simulink model "Kin3R_Giaitich"  (R2018b)
settings: Solver=VariableStepAuto  StartTime=0.0  StopTime=15  RelTol=1e-3
settings Model: Creator=ADMIN  LastModifiedBy=ADMIN

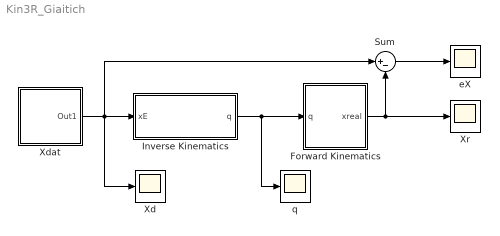
== system Kin3R_Giaitich ==
  Forward Kinematics : Subsystem
  Inverse Kinematics : Subsystem
  Sum : Sum  Inputs=|+-
  Xd : Scope
  Xdat : Subsystem
  Xr : Scope
  eX : Scope
  q : Scope
  wires:
  Xdat/1(Out1) -> Xd/1, Sum/1, Inverse Kinematics/1(xE)
  Inverse Kinematics/1(q) -> q/1, Forward Kinematics/1(q)
  Sum/1 -> eX/1
  Forward Kinematics/1(xreal) -> Xr/1, Sum/2

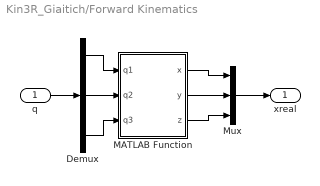
== system Kin3R_Giaitich/Forward Kinematics ==
  q : Inport
  Demux : Demux  Outputs=3
  MATLAB Function : MATLAB Function  TreatAsAtomicUnit=on
  Mux : Mux  Inputs=3
  xreal : Outport
  wires:
  Mux/1 -> xreal/1
  MATLAB Function/2(y) -> Mux/2
  MATLAB Function/1(x) -> Mux/1
  MATLAB Function/3(z) -> Mux/3
  q/1 -> Demux/1
  Demux/3 -> MATLAB Function/3(q3)
  Demux/2 -> MATLAB Function/2(q2)
  Demux/1 -> MATLAB Function/1(q1)

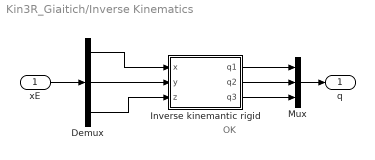
== system Kin3R_Giaitich/Inverse Kinematics ==
  note: OK
  xE : Inport
  Demux : Demux  Outputs=3
  Inverse kinemantic rigid : MATLAB Function  TreatAsAtomicUnit=on
  Mux : Mux  Inputs=3
  q : Outport
  wires:
  Mux/1 -> q/1
  Demux/1 -> Inverse kinemantic rigid/1(x)
  Demux/2 -> Inverse kinemantic rigid/2(y)
  Inverse kinemantic rigid/1(q1) -> Mux/1
  Inverse kinemantic rigid/2(q2) -> Mux/2
  xE/1 -> Demux/1
  Demux/3 -> Inverse kinemantic rigid/3(z)
  Inverse kinemantic rigid/3(q3) -> Mux/3

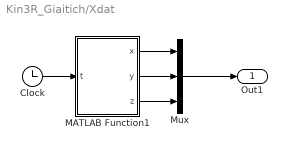
== system Kin3R_Giaitich/Xdat ==
  Clock : Clock
  MATLAB Function1 : MATLAB Function  TreatAsAtomicUnit=on
  Mux : Mux  Inputs=3
  Out1 : Outport
  wires:
  Clock/1 -> MATLAB Function1/1(t)
  Mux/1 -> Out1/1
  MATLAB Function1/1(x) -> Mux/1
  MATLAB Function1/2(y) -> Mux/2
  MATLAB Function1/3(z) -> Mux/3

== matlab function Kin3R_Giaitich/Inverse Kinematics/Inverse kinemantic rigid ==
  data: x input; q1 output; y input; q2 output; z input; q3 output
function [q1,q2,q3] = fcn(x,y,z)
%
[d1,a2,a3]=parameter();
%
q1=atan2(y,x);
%
A3=(x^2+y^2+(d1-z)^2-a2^2-a3^2)/(2*a2*a3);
q3=-acos(A3);
%
r=-sqrt(x^2+y^2);
A=a2+a3*cos(q3);
B=a3*sin(q3);
%
q2=atan2(r,z-d1)+atan2(A,B);
end

== matlab function Kin3R_Giaitich/Forward Kinematics/MATLAB Function ==
  data: x output; q1 input; y output; q2 input; q3 input; z output
function [x,y,z] = fcn(q1,q2,q3)
[d1,a2,a3]=parameter();
%% Toa do diem thao tac theo inverse(H10).D6

x=cos(q1)*(a2*cos(q2)+a3*cos(q2+q3));
y=sin(q1)*(a2*cos(q2)+a3*cos(q2+q3));
z=d1+a2*sin(q2)+a3*sin(q2+q3);

== matlab function Kin3R_Giaitich/Xdat/MATLAB Function1 ==
  data: x output; y output; t input; z output
function [x,y,z] = fcn(t)
[d1,a2,a3]=parameter();

x=0.2+0.05*cos(pi*t/4); %m
y=0.2+0.05*sin(pi*t/4); %m
z=d1*0.01*t+0.4; %m
